simulink library "lib_Convection_FCVertPlateLamConvAnalytical"  (R2015a)
settings: Solver=ode45  StartTime=0.0  StopTime=10.0  RelTol=1e-3
libraries: simulink x1
settings Model: Creator=jlkratz  LastModifiedBy=jlkratz

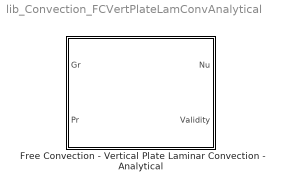
== system lib_Convection_FCVertPlateLamConvAnalytical ==
  Free Convection - Vertical Plate Laminar Convection - Analytical : Subsystem  mask(TSAT: Vertical Plate Laminar Free Convection - Analytical){}
      mask help:
      | This block estimates the average Nusselt number of free convecting flow past one side of an isothermal vertical flat plate or vertical surface. The average Nusselt number is calculated based on an analytical solution for and isothermal vertical surface in an extensive quiescent medium. Note that all fluid properrties should be evaluated at film temperature (average of the bulk fluid and surface temperatures).
      |
      | For more information see the block help menu.
      mask Help: web(which('Convection_TSAT_FCVertPlateLamConvAnalytical.html'),'-helpbrowser')

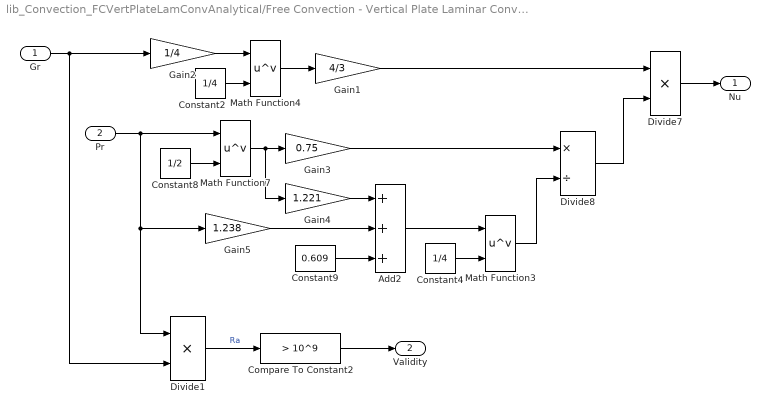
== system lib_Convection_FCVertPlateLamConvAnalytical/Free Convection - Vertical Plate Laminar Convection - Analytical ==
  Gr : Inport
  Pr : Inport  Port=2
  Add2 : Sum  Inputs=+++
  Compare To Constant2 : simulink/Logic and Bit Operations/Compare To Constant  relop=>  const=10^9  OutDataTypeStr=boolean
  Constant2 : Constant  Value=1/4
  Constant4 : Constant  Value=1/4
  Constant8 : Constant  Value=1/2
  Constant9 : Constant  Value=0.609
  Divide1 : Product  Inputs=**
  Divide7 : Product  Inputs=**
  Divide8 : Product  Inputs=*/
  Gain1 : Gain  Gain=4/3
  Gain2 : Gain  Gain=1/4
  Gain3 : Gain  Gain=0.75
  Gain4 : Gain  Gain=1.221
  Gain5 : Gain  Gain=1.238
  Math Function3 : Math  Operator=pow  SaturateOnIntegerOverflow=on
  Math Function4 : Math  Operator=pow  SaturateOnIntegerOverflow=on
  Math Function7 : Math  Operator=pow  SaturateOnIntegerOverflow=on
  Nu : Outport
  Validity : Outport  Port=2
  wires:
  Compare To Constant2/1 -> Validity/1
  Divide1/1 -> Compare To Constant2/1  "Ra"
  Divide7/1 -> Nu/1
  Divide8/1 -> Divide7/2
  Add2/1 -> Math Function3/1
  Gain5/1 -> Add2/2
  Math Function7/1 -> Gain3/1, Gain4/1
  Gain4/1 -> Add2/1
  Constant9/1 -> Add2/3
  Math Function3/1 -> Divide8/2
  Gain3/1 -> Divide8/1
  Pr/1 -> Math Function7/1, Gain5/1, Divide1/1
  Constant8/1 -> Math Function7/2
  Constant4/1 -> Math Function3/2
  Gain1/1 -> Divide7/1
  Math Function4/1 -> Gain1/1
  Gain2/1 -> Math Function4/1
  Gr/1 -> Gain2/1, Divide1/2
  Constant2/1 -> Math Function4/2
